simulink library "UXFD_Lib"  (R2016b)
settings: Solver=ode45  StartTime=0.0  StopTime=10.0  RelTol=1e-3  EnableMultiTasking=on
undefined symbols (not defined in the file): BreakpointData, BreakpointData1, BreakpointData2, BreakpointData_One_A, BreakpointData_Two_A, E2E_P01DataIDMode, E2E_P01ReceiverStatusType, EnumClass, iBit, initalValue, No_Runnable_Period, ObB_EidBsgStDerat_C, p_OVERRIDE_MASTER_SWITCH, SlDemoSign, SwitchOff_P, SwitchOn_P, Table, TableData_M, VCCTi33, VSysD_FidVehDerat1_C
libraries: simulink x28, CCMLib x11, UXFD_Lib x8, canmsglib x2, PTCC_Lib x1, hdlsllib x1
(part 2 of 7)

== system UXFD_Lib/Autosar/Dem_SetEventStatusDepPP ==
  VcEv : Inport
  EntryCond : EnablePort
  Dem_SetEventStatus : S-Function  FunctionName=Dem_SetEventStatusDep_flp  Parameters=dt  SFunctionDeploymentMode=off  EnableBusSupport=off  mask(TL_CustomCode){data={'#state',0,'#param',0,'#work',0,'#input',2,'codefile','Dem_SetEventStatusDep.c','prodcode',0,'logdata',{'plotchannels',[]},'output',{'name','$S_ok','varname','ok','type','Bool'},'input#1',{'name','$S_EventId','varname','EventId','type','UInt16'},'input#2',{'name','$S_EventStatus','varname','EventStatus','type','UInt8'},'date',735284.44087483792}, dt=-1}
      mask help:
      | TargetLink Custom Code block:
      | Allows to insert custom code into a TargetLink application.
      settings: AttributesFormatString=Dem_SetEventStatusDep  DeleteFcn=if exist('delete_tlblock','file')==2,delete_tlblock(gcbh);end  NameChangeFcn=if exist('rename_tlblock','file')==2,rename_tlblock(gcbh);end  OpenFcn=if exist('tl_open_blockdlg','file')==2,tl_open_blockdlg(gcbh);else,open_system(gcbh,'mask');end
      mask Help: eval(['tl_online_help(''Topic'',''',get_param(gcbh,'MaskType'),''')'])
      mask Display:
      | plot([-0.05, 1.05, NaN, -0.05, 1.05],[.01, .01, NaN, .99, .99])
      | ; disp('Dem_SetEventStatusDep.c');port_label('input',1,'EventId');port_label('input',2,'EventStatus');port_label('output',1,'ok');
  Pre-Passed : Constant  Value=2  mask(TL_Constant){data={'date',735284.44033693289}}
      settings: CopyFcn=if exist('tl_reset_reviewflag','file')==2,tl_reset_reviewflag(gcbh);end  DeleteFcn=if exist('delete_tlblock','file')==2,delete_tlblock(gcbh);end  NameChangeFcn=if exist('rename_tlblock','file')==2,rename_tlblock(gcbh);end  OpenFcn=if exist('tl_open_blockdlg','file')==2,tl_open_blockdlg(gcbh);else,open_system(gcbh,'parameter');end
      mask Help: eval(['if exist(''tl_online_help'',''file'') == 2, tl_online_help(''Topic'',''TL_Constant''),else, web([''jar:file:///'',matlabroot,''/help/toolbox/simulink/help.jar!/slref/' lower(get_param(gcbh,'Blocktype')) '.html''], ''-helpbrowser''),end'])
      mask Display: plot([-0.05, 1.05, NaN, -0.05, 1.05],[.01, .01, NaN, .99, .99])
  Terminator3 : Terminator
  wires:
  Dem_SetEventStatus/1 -> Terminator3/1
  VcEv/1 -> Dem_SetEventStatus/1
  Pre-Passed/1 -> Dem_SetEventStatus/2

== system UXFD_Lib/Autosar/Dem_SetEventStatusF ==
  VcEv : Inport
  EntryCond : EnablePort
  Dem_SetEventStatus : S-Function  FunctionName=Dem_SetEventStatus_flp  Parameters=dt  SFunctionDeploymentMode=off  EnableBusSupport=off  mask(TL_CustomCode){data={'#state',0,'#param',0,'#work',0,'#input',2,'codefile','Dem_SetEventStatus.c','prodcode',0,'logdata',{'plotchannels',[]},'output',{'name','$S_ok','varname','ok','type','Bool'},'input#1',{'name','$S_EventId','varname','EventId','type','UInt16'},'input#2',{'name','$S_EventStatus','varname','EventStatus','type','UInt8'},'date',735300.29239828698}, dt=-1}
      mask help:
      | TargetLink Custom Code block:
      | Allows to insert custom code into a TargetLink application.
      settings: AttributesFormatString=Dem_SetEventStatus  DeleteFcn=if exist('delete_tlblock','file')==2,delete_tlblock(gcbh);end  NameChangeFcn=if exist('rename_tlblock','file')==2,rename_tlblock(gcbh);end  OpenFcn=if exist('tl_open_blockdlg','file')==2,tl_open_blockdlg(gcbh);else,open_system(gcbh,'mask');end
      mask Help: eval(['tl_online_help(''Topic'',''',get_param(gcbh,'MaskType'),''')'])
      mask Display:
      | plot([-0.05, 1.05, NaN, -0.05, 1.05],[.01, .01, NaN, .99, .99])
      | ; disp('Dem_SetEventStatus.c');port_label('input',1,'EventId');port_label('input',2,'EventStatus');port_label('output',1,'ok');
  Failed : Constant  mask(TL_Constant){data={'date',735300.29239776626}}
      settings: CopyFcn=if exist('tl_reset_reviewflag','file')==2,tl_reset_reviewflag(gcbh);end  DeleteFcn=if exist('delete_tlblock','file')==2,delete_tlblock(gcbh);end  NameChangeFcn=if exist('rename_tlblock','file')==2,rename_tlblock(gcbh);end  OpenFcn=if exist('tl_open_blockdlg','file')==2,tl_open_blockdlg(gcbh);else,open_system(gcbh,'parameter');end
      mask Help: eval(['if exist(''tl_online_help'',''file'') == 2, tl_online_help(''Topic'',''TL_Constant''),else, web([''jar:file:///'',matlabroot,''/help/toolbox/simulink/help.jar!/slref/' lower(get_param(gcbh,'Blocktype')) '.html''], ''-helpbrowser''),end'])
      mask Display: plot([-0.05, 1.05, NaN, -0.05, 1.05],[.01, .01, NaN, .99, .99])
  Terminator3 : Terminator
  wires:
  Dem_SetEventStatus/1 -> Terminator3/1
  VcEv/1 -> Dem_SetEventStatus/1
  Failed/1 -> Dem_SetEventStatus/2

== system UXFD_Lib/Autosar/Dem_SetEventStatusP ==
  VcEv : Inport
  EntryCond : EnablePort
  Dem_SetEventStatus : S-Function  FunctionName=Dem_SetEventStatus_flp  Parameters=dt  SFunctionDeploymentMode=off  EnableBusSupport=off  mask(TL_CustomCode){data={'#state',0,'#param',0,'#work',0,'#input',2,'codefile','Dem_SetEventStatus.c','prodcode',0,'logdata',{'plotchannels',[]},'output',{'name','$S_ok','varname','ok','type','Bool'},'input#1',{'name','$S_EventId','varname','EventId','type','UInt16'},'input#2',{'name','$S_EventStatus','varname','EventStatus','type','UInt8'},'date',735300.29239747685}, dt=-1}
      mask help:
      | TargetLink Custom Code block:
      | Allows to insert custom code into a TargetLink application.
      settings: AttributesFormatString=Dem_SetEventStatus  DeleteFcn=if exist('delete_tlblock','file')==2,delete_tlblock(gcbh);end  NameChangeFcn=if exist('rename_tlblock','file')==2,rename_tlblock(gcbh);end  OpenFcn=if exist('tl_open_blockdlg','file')==2,tl_open_blockdlg(gcbh);else,open_system(gcbh,'mask');end
      mask Help: eval(['tl_online_help(''Topic'',''',get_param(gcbh,'MaskType'),''')'])
      mask Display:
      | plot([-0.05, 1.05, NaN, -0.05, 1.05],[.01, .01, NaN, .99, .99])
      | ; disp('Dem_SetEventStatus.c');port_label('input',1,'EventId');port_label('input',2,'EventStatus');port_label('output',1,'ok');
  Passed : Constant  Value=0  mask(TL_Constant){data={'date',735300.29239693284}}
      settings: CopyFcn=if exist('tl_reset_reviewflag','file')==2,tl_reset_reviewflag(gcbh);end  DeleteFcn=if exist('delete_tlblock','file')==2,delete_tlblock(gcbh);end  NameChangeFcn=if exist('rename_tlblock','file')==2,rename_tlblock(gcbh);end  OpenFcn=if exist('tl_open_blockdlg','file')==2,tl_open_blockdlg(gcbh);else,open_system(gcbh,'parameter');end
      mask Help: eval(['if exist(''tl_online_help'',''file'') == 2, tl_online_help(''Topic'',''TL_Constant''),else, web([''jar:file:///'',matlabroot,''/help/toolbox/simulink/help.jar!/slref/' lower(get_param(gcbh,'Blocktype')) '.html''], ''-helpbrowser''),end'])
      mask Display: plot([-0.05, 1.05, NaN, -0.05, 1.05],[.01, .01, NaN, .99, .99])
  Terminator3 : Terminator
  wires:
  Passed/1 -> Dem_SetEventStatus/2
  VcEv/1 -> Dem_SetEventStatus/1
  Dem_SetEventStatus/1 -> Terminator3/1

== system UXFD_Lib/Autosar/Dem_SetEventStatusPF ==
  VcEv : Inport
  EntryCond : EnablePort
  Dem_SetEventStatus : S-Function  FunctionName=Dem_SetEventStatus_flp  Parameters=dt  SFunctionDeploymentMode=off  EnableBusSupport=off  mask(TL_CustomCode){data={'#state',0,'#param',0,'#work',0,'#input',2,'codefile','Dem_SetEventStatus.c','prodcode',0,'logdata',{'plotchannels',[]},'output',{'name','$S_ok','varname','ok','type','Bool'},'input#1',{'name','$S_EventId','varname','EventId','type','UInt16'},'input#2',{'name','$S_EventStatus','varname','EventStatus','type','UInt8'},'date',735300.29239666671}, dt=-1}
      mask help:
      | TargetLink Custom Code block:
      | Allows to insert custom code into a TargetLink application.
      settings: AttributesFormatString=Dem_SetEventStatus  DeleteFcn=if exist('delete_tlblock','file')==2,delete_tlblock(gcbh);end  NameChangeFcn=if exist('rename_tlblock','file')==2,rename_tlblock(gcbh);end  OpenFcn=if exist('tl_open_blockdlg','file')==2,tl_open_blockdlg(gcbh);else,open_system(gcbh,'mask');end
      mask Help: eval(['tl_online_help(''Topic'',''',get_param(gcbh,'MaskType'),''')'])
      mask Display:
      | plot([-0.05, 1.05, NaN, -0.05, 1.05],[.01, .01, NaN, .99, .99])
      | ; disp('Dem_SetEventStatus.c');port_label('input',1,'EventId');port_label('input',2,'EventStatus');port_label('output',1,'ok');
  Pre-Failed : Constant  Value=3  mask(TL_Constant){data={'date',735300.2923961574}}
      settings: CopyFcn=if exist('tl_reset_reviewflag','file')==2,tl_reset_reviewflag(gcbh);end  DeleteFcn=if exist('delete_tlblock','file')==2,delete_tlblock(gcbh);end  NameChangeFcn=if exist('rename_tlblock','file')==2,rename_tlblock(gcbh);end  OpenFcn=if exist('tl_open_blockdlg','file')==2,tl_open_blockdlg(gcbh);else,open_system(gcbh,'parameter');end
      mask Help: eval(['if exist(''tl_online_help'',''file'') == 2, tl_online_help(''Topic'',''TL_Constant''),else, web([''jar:file:///'',matlabroot,''/help/toolbox/simulink/help.jar!/slref/' lower(get_param(gcbh,'Blocktype')) '.html''], ''-helpbrowser''),end'])
      mask Display: plot([-0.05, 1.05, NaN, -0.05, 1.05],[.01, .01, NaN, .99, .99])
  Terminator3 : Terminator
  wires:
  Pre-Failed/1 -> Dem_SetEventStatus/2
  VcEv/1 -> Dem_SetEventStatus/1
  Dem_SetEventStatus/1 -> Terminator3/1

== system UXFD_Lib/Autosar/Dem_SetEventStatusPP ==
  VcEv : Inport
  EntryCond : EnablePort
  Dem_SetEventStatus : S-Function  FunctionName=Dem_SetEventStatus_flp  Parameters=dt  SFunctionDeploymentMode=off  EnableBusSupport=off  mask(TL_CustomCode){data={'#state',0,'#param',0,'#work',0,'#input',2,'codefile','Dem_SetEventStatus.c','prodcode',0,'logdata',{'plotchannels',[]},'output',{'name','$S_ok','varname','ok','type','Bool'},'input#1',{'name','$S_EventId','varname','EventId','type','UInt16'},'input#2',{'name','$S_EventStatus','varname','EventStatus','type','UInt8'},'date',735300.29239586811}, dt=-1}
      mask help:
      | TargetLink Custom Code block:
      | Allows to insert custom code into a TargetLink application.
      settings: AttributesFormatString=Dem_SetEventStatus  DeleteFcn=if exist('delete_tlblock','file')==2,delete_tlblock(gcbh);end  NameChangeFcn=if exist('rename_tlblock','file')==2,rename_tlblock(gcbh);end  OpenFcn=if exist('tl_open_blockdlg','file')==2,tl_open_blockdlg(gcbh);else,open_system(gcbh,'mask');end
      mask Help: eval(['tl_online_help(''Topic'',''',get_param(gcbh,'MaskType'),''')'])
      mask Display:
      | plot([-0.05, 1.05, NaN, -0.05, 1.05],[.01, .01, NaN, .99, .99])
      | ; disp('Dem_SetEventStatus.c');port_label('input',1,'EventId');port_label('input',2,'EventStatus');port_label('output',1,'ok');
  Pre-Passed : Constant  Value=2  mask(TL_Constant){data={'date',735300.29237822921}}
      settings: CopyFcn=if exist('tl_reset_reviewflag','file')==2,tl_reset_reviewflag(gcbh);end  DeleteFcn=if exist('delete_tlblock','file')==2,delete_tlblock(gcbh);end  NameChangeFcn=if exist('rename_tlblock','file')==2,rename_tlblock(gcbh);end  OpenFcn=if exist('tl_open_blockdlg','file')==2,tl_open_blockdlg(gcbh);else,open_system(gcbh,'parameter');end
      mask Help: eval(['if exist(''tl_online_help'',''file'') == 2, tl_online_help(''Topic'',''TL_Constant''),else, web([''jar:file:///'',matlabroot,''/help/toolbox/simulink/help.jar!/slref/' lower(get_param(gcbh,'Blocktype')) '.html''], ''-helpbrowser''),end'])
      mask Display: plot([-0.05, 1.05, NaN, -0.05, 1.05],[.01, .01, NaN, .99, .99])
  Terminator3 : Terminator
  wires:
  Dem_SetEventStatus/1 -> Terminator3/1
  VcEv/1 -> Dem_SetEventStatus/1
  Pre-Passed/1 -> Dem_SetEventStatus/2

== system UXFD_Lib/Autosar/E2E_P01Protect ==
  DataLength : Inport
  DataID : Inport  Port=2
  Vmc_Out_BrkActrCtrlModForMinTqReq : Inport  Port=3
  Vmc_Out_BrkTqGrdtNegMinReq : Inport  Port=4
  Vmc_Out_BrkTqGrdtPosMinReq : Inport  Port=5
  Vmc_Out_BrkTqMinReq : Inport  Port=6
  E2E_P01Protect : Subsystem  TreatAsAtomicUnit=on
  Selector : Selector  InputPortWidth=9  IndexOptions=Index vector (dialog)  Indices=[1]  OutputSizes=1
  Selector1 : Selector  InputPortWidth=9  IndexOptions=Index vector (dialog)  Indices=[2]  OutputSizes=1
  Unit Delay1 : UnitDelay  SampleTime=-1
  Unit Delay2 : UnitDelay  SampleTime=-1
  E2E_P01Protect_ReturnType : Outport
  RollingCounter : Outport  Port=2
  CheckSum : Outport  Port=3
  wires:
  Selector/1 -> Unit Delay1/1, CheckSum/1
  Selector1/1 -> RollingCounter/1, Unit Delay2/1
  E2E_P01Protect/2(Data_pu8) -> Selector1/1, Selector/1
  DataLength/1 -> E2E_P01Protect/1(DataLength)
  DataID/1 -> E2E_P01Protect/2(DataID)
  E2E_P01Protect/1(E2E_P01Protect_ReturnType) -> E2E_P01Protect_ReturnType/1
  Unit Delay1/1 -> E2E_P01Protect/8(CheckSum_In)
  Unit Delay2/1 -> E2E_P01Protect/7(RollingCounter_In)
  Vmc_Out_BrkTqMinReq/1 -> E2E_P01Protect/6(Vmc_Out_BrkTqMinReq)
  Vmc_Out_BrkTqGrdtPosMinReq/1 -> E2E_P01Protect/5(Vmc_Out_BrkTqGrdtPosMinReq)
  Vmc_Out_BrkTqGrdtNegMinReq/1 -> E2E_P01Protect/4(Vmc_Out_BrkTqGrdtNegMinReq)
  Vmc_Out_BrkActrCtrlModForMinTqReq/1 -> E2E_P01Protect/3(Vmc_Out_BrkActrCtrlModForMinTqReq)

== system UXFD_Lib/Autosar/E2E_P01_Check ==
  AccrPedlNotCmpl_IsUpdated : Inport  OutDataTypeStr=boolean
  CheckSum : Inport  Port=2
  RollingCounter : Inport  Port=3
  AccrPedlNotCmpl_Psd : Inport  Port=4
  AccrPedlNotCmpl_PsdSts : Inport  Port=5
  DataID_ID : Constant  Value=205  OutDataTypeStr=uint16
  DataLength : Constant  Value=32  OutDataTypeStr=uint16
  E2E_Check : Subsystem
  E2E_check_OK : Outport
  wires:
  DataLength/1 -> E2E_Check/1(DataLength)
  DataID_ID/1 -> E2E_Check/2(DataID)
  AccrPedlNotCmpl_IsUpdated/1 -> E2E_Check/3(AccrPedlNotCmpl_IsUpdated)
  CheckSum/1 -> E2E_Check/4(CheckSum)
  RollingCounter/1 -> E2E_Check/5(RollingCounter)
  E2E_Check/1(CRC_Valid) -> E2E_check_OK/1
  AccrPedlNotCmpl_Psd/1 -> E2E_Check/6(AccrPedlNotCmpl_Psd)
  AccrPedlNotCmpl_PsdSts/1 -> E2E_Check/7(AccrPedlNotCmpl_PsdSts)

== system UXFD_Lib/Autosar/FiM_GetFunctionPermission ==
  note: A fix for setting the correct data type in simulink.
      | The data type set in TL does not seem to propagete to
      | the simulink block.
  VcFi : Inport
  EntryCond : EnablePort
  Data Type Conversion : DataTypeConversion  OutDataTypeStr=boolean
  FiM_GetFunctionPermission : S-Function  Description=I: FID, O1 = ok, O2 = Permission  FunctionName=FiM_GetFunctionPermission_flp  Parameters=dt  SFunctionDeploymentMode=off  EnableBusSupport=off  mask(TL_CustomCode){data={'#state',0,'#param',0,'#work',0,'#output',2,'#logdata',2,'codefile','FiM_GetFunctionPermission.c','prodcode',0,'logdata#1',{'plotchannels',[]},'logdata#2',{'plotchannels',[]},'output#1',{'name','$S_ok','varname','ok','type','Bool'},'output#2',{'name','$S_perm','varname','permission','type','Bool'},'input',{'name','$S_FID','varname','FID','type','UInt16'},'date',736012.81500542827}, dt=-1}
      mask help:
      | TargetLink Custom Code block:
      | Allows to insert custom code into a TargetLink application.
      settings: AttributesFormatString=FiM_GetFunctionPermission  DeleteFcn=if exist('delete_tlblock','file')==2,delete_tlblock(gcbh);end  NameChangeFcn=if exist('rename_tlblock','file')==2,rename_tlblock(gcbh);end  OpenFcn=if exist('tl_open_blockdlg','file')==2,tl_open_blockdlg(gcbh);else,open_system(gcbh,'mask');end
      mask Help: eval(['tl_online_help(''Topic'',''',get_param(gcbh,'MaskType'),''')'])
      mask Display:
      | plot([-0.05, 1.05, NaN, -0.05, 1.05],[.01, .01, NaN, .99, .99])
      | ; disp('FiM_GetFunctionPermission.c');port_label('input',1,'FID');port_label('output',1,'ok');port_label('output',2,'permission');
  Terminator4 : Terminator
  Perm : Outport
  wires:
  FiM_GetFunctionPermission/2 -> Data Type Conversion/1
  FiM_GetFunctionPermission/1 -> Terminator4/1
  VcFi/1 -> FiM_GetFunctionPermission/1
  Data Type Conversion/1 -> Perm/1

== system UXFD_Lib/Autosar/NamedConstant ==
  Constant : Constant  Value=0  mask(TL_Constant){data={'output',{'name','$E(const_name)','class','EXTERN_GLOBAL_ALIAS','type','UInt16'},'date',735602.50771956018}}
      settings: AttributesFormatString=%<const_name>  CopyFcn=if exist('tl_reset_reviewflag') == 2, tl_reset_reviewflag(gcbh); end  DeleteFcn=if exist('delete_tlblock','file')==2,delete_tlblock(gcbh);end  NameChangeFcn=if exist('rename_tlblock','file')==2,rename_tlblock(gcbh);end  OpenFcn=if exist('tl_open_blockdlg','file')==2,tl_open_blockdlg(gcbh);else,open_system(gcbh,'parameter');end
      mask Help: eval(['if exist(''tl_online_help'',''file'') == 2, tl_online_help(''Topic'',''TL_Constant''),else, web([''jar:file:///'',matlabroot,''/help/toolbox/simulink/help.jar!/slref/' lower(get_param(gcbh,'Blocktype')) '.html''], ''-helpbrowser''),end'])
      mask Display: plot([-0.05, 1.05, NaN, -0.05, 1.05],[.01, .01, NaN, .99, .99])
  Perm : Outport
  wires:
  Constant/1 -> Perm/1

== system UXFD_Lib/Autosar/xbackground4 ==

== system UXFD_Lib/Autosar/xbackground5 ==

== system UXFD_Lib/CCM/1-D LookupTable ==
  XAxis : Inport
  1-D Lookup Table : Lookup_n-D  NumberOfTableDimensions=1  BreakpointsForDimension1=BreakpointsXAxis  BreakpointsForDimension1DataTypeStr=BreakpointsXAxisDataType  Table=TableData  TableDataTypeStr=TableDataDataType  ExtrapMethod=Clip  UseLastTableValue=on  OutDataTypeStr=TableDataDataType  SaturateOnIntegerOverflow=on
  Out : Outport
  wires:
  1-D Lookup Table/1 -> Out/1
  XAxis/1 -> 1-D Lookup Table/1

== system UXFD_Lib/CCM/2-D LookupTable ==
  XAxis : Inport
  YAxis : Inport  Port=2
  2-D Lookup Table : Lookup_n-D  BreakpointsForDimension1=BreakpointsYAxis  BreakpointsForDimension2=BreakpointsXAxis  BreakpointsForDimension1DataTypeStr=BreakpointsYAxisDataType  BreakpointsForDimension2DataTypeStr=BreakpointsXAxisDataType  Table=TableData  TableDataTypeStr=TableDataDataType  ExtrapMethod=Clip  UseLastTableValue=on  OutDataTypeStr=TableDataDataType  SaturateOnIntegerOverflow=on
  Out : Outport
  wires:
  XAxis/1 -> 2-D Lookup Table/2
  YAxis/1 -> 2-D Lookup Table/1
  2-D Lookup Table/1 -> Out/1

== system UXFD_Lib/CCM/CompareToEnum ==
  u : Inport
  Compare : RelationalOperator  Operator===  OutDataTypeStr=boolean  RndMeth=Nearest  InputSameDT=on
  Constant : Constant  DisableCoverage=on  Value=const  OutDataTypeStr=Inherit: Inherit via back propagation
  y : Outport
  wires:
  u/1 -> Compare/1
  Constant/1 -> Compare/2
  Compare/1 -> y/1

== system UXFD_Lib/CCM/Conversion ==
  In : Inport
  Data Type Conversion : DataTypeConversion  OutDataTypeStr=outputDataType  SaturateOnIntegerOverflow=on
  Out : Outport
  wires:
  In/1 -> Data Type Conversion/1
  Data Type Conversion/1 -> Out/1

== system UXFD_Lib/CCM/Counter ==
  note: CounterRunning
  Start : Inport  OutDataTypeStr=boolean
  Reset : Inport  Port=2  OutDataTypeStr=boolean
  IC : Constant  Value=0  OutDataTypeStr=VCCUInt32  SampleTime=-1
  Increment : Constant  OutDataTypeStr=VCCUInt32  SampleTime=-1
  Logical Operator : Logic  AllPortsSameDT=off  OutDataTypeStr=boolean
  Logical Operator1 : Logic  Operator=NOT  AllPortsSameDT=off  OutDataTypeStr=boolean
  Logical Operator2 : Logic  Operator=OR  AllPortsSameDT=off  OutDataTypeStr=boolean
  StopCounter : Constant  Value=0  OutDataTypeStr=VCCUInt32  SampleTime=-1
  Sum : Sum  OutDataTypeStr=VCCUInt32  SaturateOnIntegerOverflow=on
  Switch : Switch  Criteria=u2 ~= 0  SaturateOnIntegerOverflow=on
  Unit Delay External IC : simulink/Additional Math & Discrete/Additional Discrete/Unit Delay External IC  tsamp=-1
  Unit Delay Resettable External IC : CCMLib/Unit Delay Resettable External IC  dataType=VCCUInt32
  false : Constant  Value=false  OutDataTypeStr=boolean  SampleTime=-1
  Value : Outport  OutDataTypeStr=VCCUInt32
  wires:
  StopCounter/1 -> Switch/3
  Increment/1 -> Switch/1
  Switch/1 -> Sum/2
  Reset/1 -> Unit Delay Resettable External IC/3, Logical Operator1/1
  Sum/1 -> Unit Delay Resettable External IC/1
  Unit Delay Resettable External IC/1 -> Value/1, Sum/1
  IC/1 -> Unit Delay Resettable External IC/2
  Unit Delay External IC/1 -> Logical Operator2/1
  Start/1 -> Logical Operator2/2
  Logical Operator/1 -> Unit Delay External IC/1, Switch/2
  false/1 -> Unit Delay External IC/2
  Logical Operator2/1 -> Logical Operator/1
  Logical Operator1/1 -> Logical Operator/2

== system UXFD_Lib/CCM/Counter Holdable ==
  note: CounterRunning
  Start : Inport  OutDataTypeStr=boolean
  Hold : Inport  Port=2  OutDataTypeStr=boolean
  Reset : Inport  Port=3  OutDataTypeStr=boolean
  IC : Constant  Value=0  OutDataTypeStr=VCCUInt32  SampleTime=-1
  Increment : Constant  OutDataTypeStr=VCCUInt32  SampleTime=-1
  Logical Operator : Logic  AllPortsSameDT=off  OutDataTypeStr=boolean
  Logical Operator1 : Logic  Operator=NOT  AllPortsSameDT=off  OutDataTypeStr=boolean
  Logical Operator2 : Logic  Operator=OR  AllPortsSameDT=off  OutDataTypeStr=boolean
  StopCounter : Constant  Value=0  OutDataTypeStr=VCCUInt32  SampleTime=-1
  Sum : Sum  OutDataTypeStr=VCCUInt32  SaturateOnIntegerOverflow=on
  Switch : Switch  Criteria=u2 ~= 0  SaturateOnIntegerOverflow=on
  Unit Delay External IC : simulink/Additional Math & Discrete/Additional Discrete/Unit Delay External IC  tsamp=-1
  Unit Delay Resettable External IC1 : CCMLib/Unit Delay Resettable External IC  dataType=VCCUInt32
  false : Constant  Value=false  OutDataTypeStr=boolean  SampleTime=-1
  Value : Outport  OutDataTypeStr=VCCUInt32
  wires:
  IC/1 -> Unit Delay Resettable External IC1/2
  Unit Delay Resettable External IC1/1 -> Sum/1, Value/1
  Sum/1 -> Unit Delay Resettable External IC1/1
  Logical Operator1/1 -> Logical Operator/2
  Hold/1 -> Logical Operator1/1
  Logical Operator2/1 -> Logical Operator/1
  false/1 -> Unit Delay External IC/2
  Logical Operator/1 -> Switch/2, Unit Delay External IC/1
  Start/1 -> Logical Operator2/2
  Unit Delay External IC/1 -> Logical Operator2/1
  Reset/1 -> Unit Delay Resettable External IC1/3
  Switch/1 -> Sum/2
  Increment/1 -> Switch/1
  StopCounter/1 -> Switch/3

== system UXFD_Lib/CCM/LowPass filter ==
  note: filtered signal
  note: NOTE!
      | LPF_Time_Constant must be greater
      | or equal to the Sample_Time
  U : Inport  OutDataTypeStr=InputOutputDataType
  FilCon : Inport  Port=2  OutDataTypeStr=FilterConstantDataType
  Constant : Constant  OutDataTypeStr=single  SampleTime=-1
  Data Type Conversion1 : DataTypeConversion  OutDataTypeStr=single  RndMeth=Round  SaturateOnIntegerOverflow=on
  MinMax : MinMax  Function=max  Inputs=2  OutDataTypeStr=single  SaturateOnIntegerOverflow=on
  OutputDataType : DataTypeConversion  OutDataTypeStr=InputOutputDataType  RndMeth=Round  SaturateOnIntegerOverflow=on
  Product1 : Product  Inputs=*/  OutDataTypeStr=single  SaturateOnIntegerOverflow=on
  Product2 : Product  OutDataTypeStr=single  SaturateOnIntegerOverflow=on
  Product3 : Product  OutDataTypeStr=single  SaturateOnIntegerOverflow=on
  RunnablePeriod : Constant  Value=RunnablePeriod  OutDataTypeStr=single  SampleTime=-1
  Sum : Sum  Inputs=+-  OutDataTypeStr=single  SaturateOnIntegerOverflow=on
  Sum1 : Sum  OutDataTypeStr=single  SaturateOnIntegerOverflow=on
  Unit Delay External IC : CCMLib/Unit Delay External IC  dataType=single
  Y : Outport  OutDataTypeStr=InputOutputDataType
  wires:
  FilCon/1 -> MinMax/2
  MinMax/1 -> Product1/2
  OutputDataType/1 -> Y/1
  U/1 -> Data Type Conversion1/1
  RunnablePeriod/1 -> MinMax/1, Product1/1
  Product2/1 -> Sum1/2
  Sum1/1 -> Unit Delay External IC/1, OutputDataType/1
  Unit Delay External IC/1 -> Product2/2
  Product3/1 -> Sum1/1
  Sum/1 -> Product2/1
  Product1/1 -> Product3/2, Sum/2
  Data Type Conversion1/1 -> Unit Delay External IC/2, Product3/1
  Constant/1 -> Sum/1

== system UXFD_Lib/CCM/LowPass filter Resettable ==
  note: NOTE!
      | LPF_Time_Constant must be greater
      | or equal to the Sample_Time
  note: filtered signal
  U : Inport  OutDataTypeStr=InputOutputDataType
  FilCon : Inport  Port=2  OutDataTypeStr=FilterConstantDataType
  Rst : Inport  Port=3  OutDataTypeStr=boolean
  Constant : Constant  OutDataTypeStr=single  SampleTime=-1
  Data Type Conversion1 : DataTypeConversion  OutDataTypeStr=single  SaturateOnIntegerOverflow=on
  MinMax : MinMax  Function=max  Inputs=2  OutDataTypeStr=single  SaturateOnIntegerOverflow=on
  OutputDataType : DataTypeConversion  OutDataTypeStr=InputOutputDataType  RndMeth=Round  SaturateOnIntegerOverflow=on
  Product1 : Product  Inputs=*/  OutDataTypeStr=single  SaturateOnIntegerOverflow=on  RndMeth=Zero
  Product2 : Product  OutDataTypeStr=single  SaturateOnIntegerOverflow=on
  Product3 : Product  OutDataTypeStr=single  SaturateOnIntegerOverflow=on
  RunnablePeriod : Constant  Value=RunnablePeriod  OutDataTypeStr=single  SampleTime=-1
  Sum : Sum  Inputs=+-  OutDataTypeStr=single  SaturateOnIntegerOverflow=on
  Sum1 : Sum  OutDataTypeStr=single  SaturateOnIntegerOverflow=on
  Unit Delay Resettable External IC boolean controlled : Subsystem  mask(Unit Delay Resettable External Initial Condition (boolean)){dt=single, UnitDelayInitCondition=0}
      mask prompts: dt "Data type in/out"; UnitDelayInitCondition "Internal unit delay block initial condition:"
      mask help:
      | This is the same block as the Simulink standard, except all fix point
      | data-types have been changed to booleans.
      | The internal unit delay block can often be kept as 0, unless the input/output signal is of ENUM type.
      | Made by Niklas Magnusson (nmagnus3).
      | NGCC
      mask Display: dpoly(1,[1 0],'z')
  Y : Outport  OutDataTypeStr=InputOutputDataType
  wires:
  Constant/1 -> Sum/1
  Data Type Conversion1/1 -> Product3/1, Unit Delay Resettable External IC boolean controlled/3(IC)
  Product1/1 -> Sum/2, Product3/2
  Sum/1 -> Product2/1
  Product3/1 -> Sum1/1
  Unit Delay Resettable External IC boolean controlled/1(y) -> Product2/2
  Sum1/1 -> OutputDataType/1, Unit Delay Resettable External IC boolean controlled/1(u)
  Product2/1 -> Sum1/2
  RunnablePeriod/1 -> Product1/1, MinMax/1
  U/1 -> Data Type Conversion1/1
  OutputDataType/1 -> Y/1
  Rst/1 -> Unit Delay Resettable External IC boolean controlled/2(R)
  MinMax/1 -> Product1/2
  FilCon/1 -> MinMax/2

== system UXFD_Lib/CCM/LowPass filter IC ==
  note: filtered signal
  note: NOTE!
      | LPF_Time_Constant must be greater
      | or equal to the Sample_Time
  U : Inport  OutDataTypeStr=InputOutputDataType
  IC : Inport  Port=2  OutDataTypeStr=InputOutputDataType
  FilCon : Inport  Port=3  OutDataTypeStr=FilterConstantDataType
  Constant : Constant  OutDataTypeStr=single  SampleTime=-1
  Data Type Conversion1 : DataTypeConversion  OutDataTypeStr=single  RndMeth=Round  SaturateOnIntegerOverflow=on
  Data Type Conversion2 : DataTypeConversion  OutDataTypeStr=single  RndMeth=Round  SaturateOnIntegerOverflow=on
  EnableIC : Constant  Value=true  OutDataTypeStr=boolean  SampleTime=-1
  MinMax : MinMax  Function=max  Inputs=2  OutDataTypeStr=single  SaturateOnIntegerOverflow=on
  OutputDataType : DataTypeConversion  OutDataTypeStr=InputOutputDataType  RndMeth=Round  SaturateOnIntegerOverflow=on
  Product1 : Product  Inputs=*/  OutDataTypeStr=single  SaturateOnIntegerOverflow=on
  Product2 : Product  OutDataTypeStr=single  SaturateOnIntegerOverflow=on
  Product3 : Product  OutDataTypeStr=single  SaturateOnIntegerOverflow=on
  RunnablePeriod : Constant  Value=RunnablePeriod  OutDataTypeStr=single  SampleTime=-1
  Sum : Sum  Inputs=+-  OutDataTypeStr=single  SaturateOnIntegerOverflow=on
  Sum1 : Sum  OutDataTypeStr=single  SaturateOnIntegerOverflow=on
  Switch : Switch  Criteria=u2 ~= 0  SaturateOnIntegerOverflow=on
  Unit Delay : UnitDelay  InitialCondition=false  SampleTime=-1
      settings: AttributesFormatString=X0=%<X0>
  Unit Delay External IC : CCMLib/Unit Delay External IC  dataType=single
  Y : Outport  OutDataTypeStr=InputOutputDataType
  wires:
  EnableIC/1 -> Unit Delay/1
  Unit Delay/1 -> Switch/2
  Switch/1 -> OutputDataType/1
  FilCon/1 -> MinMax/2
  MinMax/1 -> Product1/2
  OutputDataType/1 -> Y/1
  U/1 -> Data Type Conversion1/1
  RunnablePeriod/1 -> MinMax/1, Product1/1
  Product2/1 -> Sum1/2
  Sum1/1 -> Switch/1, Unit Delay External IC/1
  Unit Delay External IC/1 -> Product2/2
  Product3/1 -> Sum1/1
  Sum/1 -> Product2/1
  Product1/1 -> Product3/2, Sum/2
  Data Type Conversion1/1 -> Product3/1
  Constant/1 -> Sum/1
  IC/1 -> Data Type Conversion2/1
  Data Type Conversion2/1 -> Switch/3, Unit Delay External IC/2

== system UXFD_Lib/CCM/LowPass filter IC Resettable ==
  note: filtered signal
  note: NOTE!
      | LPF_Time_Constant must be greater
      | or equal to the Sample_Time
  U : Inport  OutDataTypeStr=InputOutputDataType
  IC : Inport  Port=2  OutDataTypeStr=InputOutputDataType
  FilCon : Inport  Port=3  OutDataTypeStr=FilterConstantDataType
  Rst : Inport  Port=4  OutDataTypeStr=boolean
  Constant : Constant  OutDataTypeStr=single  SampleTime=-1
  Data Type Conversion1 : DataTypeConversion  OutDataTypeStr=single  SaturateOnIntegerOverflow=on
  Data Type Conversion2 : DataTypeConversion  OutDataTypeStr=single  SaturateOnIntegerOverflow=on
  DisableIC : Constant  Value=false  OutDataTypeStr=boolean  SampleTime=-1
  Logical Operator : Logic  Operator=OR  AllPortsSameDT=off  OutDataTypeStr=boolean
  MinMax : MinMax  Function=max  Inputs=2  OutDataTypeStr=single  SaturateOnIntegerOverflow=on
  OutputDataType : DataTypeConversion  OutDataTypeStr=InputOutputDataType  RndMeth=Round  SaturateOnIntegerOverflow=on
  Product1 : Product  Inputs=*/  OutDataTypeStr=single  SaturateOnIntegerOverflow=on  RndMeth=Zero
  Product2 : Product  OutDataTypeStr=single  SaturateOnIntegerOverflow=on
  Product3 : Product  OutDataTypeStr=single  SaturateOnIntegerOverflow=on
  RunnablePeriod : Constant  Value=RunnablePeriod  OutDataTypeStr=single  SampleTime=-1
  Sum : Sum  Inputs=+-  OutDataTypeStr=single  SaturateOnIntegerOverflow=on
  Sum1 : Sum  OutDataTypeStr=single  SaturateOnIntegerOverflow=on
  Switch : Switch  Criteria=u2 ~= 0  SaturateOnIntegerOverflow=on
  Unit Delay : UnitDelay  InitialCondition=true  SampleTime=-1
      settings: AttributesFormatString=X0=%<X0>
  Unit Delay Resettable External IC boolean controlled : Subsystem  mask(Unit Delay Resettable External Initial Condition (boolean)){dt=single, UnitDelayInitCondition=0}
      mask prompts: dt "Data type in/out"; UnitDelayInitCondition "Internal unit delay block initial condition:"
      mask help:
      | This is the same block as the Simulink standard, except all fix point
      | data-types have been changed to booleans.
      | The internal unit delay block can often be kept as 0, unless the input/output signal is of ENUM type.
      | Made by Niklas Magnusson (nmagnus3).
      | NGCC
      mask Display: dpoly(1,[1 0],'z')
  Y : Outport  OutDataTypeStr=InputOutputDataType
  wires:
  Logical Operator/1 -> Switch/2
  Unit Delay/1 -> Logical Operator/1
  DisableIC/1 -> Unit Delay/1
  Switch/1 -> OutputDataType/1
  Data Type Conversion2/1 -> Switch/1, Unit Delay Resettable External IC boolean controlled/3(IC)
  IC/1 -> Data Type Conversion2/1
  FilCon/1 -> MinMax/2
  MinMax/1 -> Product1/2
  Rst/1 -> Logical Operator/2, Unit Delay Resettable External IC boolean controlled/2(R)
  OutputDataType/1 -> Y/1
  U/1 -> Data Type Conversion1/1
  RunnablePeriod/1 -> MinMax/1, Product1/1
  Product2/1 -> Sum1/2
  Sum1/1 -> Switch/3, Unit Delay Resettable External IC boolean controlled/1(u)
  Unit Delay Resettable External IC boolean controlled/1(y) -> Product2/2
  Product3/1 -> Sum1/1
  Sum/1 -> Product2/1
  Product1/1 -> Product3/2, Sum/2
  Data Type Conversion1/1 -> Product3/1
  Constant/1 -> Sum/1

== system UXFD_Lib/CCM/NonZero Division ==
  note: Data type conversion blocks are used to avoid error
      | when using unary minus on an unsigned data type.
  num : Inport  OutDataTypeStr=dataTypeNum
  denom : Inport  Port=2  OutDataTypeStr=dataTypeDen
  Constant1 : Constant  Value=0  OutDataTypeStr=dataTypeDen  SampleTime=-1
  Constant2 : Constant  Value=dataTypeSlope  OutDataTypeStr=dataTypeDen  SampleTime=-1
  Conversion2 : CCMLib/Conversion  outputDataType=single
  Conversion3 : CCMLib/Conversion  outputDataType=dataTypeDen
  Divide : Product  Inputs=*/  OutDataTypeStr=dataTypeOut  SaturateOnIntegerOverflow=on  RndMeth=Zero
  MinMax : MinMax  Inputs=2  OutDataTypeStr=dataTypeDen  RndMeth=Zero  SaturateOnIntegerOverflow=on
  MinMax1 : MinMax  Function=max  Inputs=2  OutDataTypeStr=dataTypeDen  RndMeth=Zero  SaturateOnIntegerOverflow=on
  Relational Operator1 : RelationalOperator  OutDataTypeStr=boolean  RndMeth=Nearest
  Switch2 : Switch  Criteria=u2 ~= 0  RndMeth=Zero  SaturateOnIntegerOverflow=on
  Unary Minus1 : UnaryMinus  SaturateOnIntegerOverflow=on
  y : Outport  OutDataTypeStr=dataTypeOut
  wires:
  Conversion3/1 -> MinMax/2
  Switch2/1 -> Divide/2
  Conversion2/1 -> Unary Minus1/1
  Constant2/1 -> MinMax1/2, Conversion2/1
  Unary Minus1/1 -> Conversion3/1
  MinMax/1 -> Switch2/3
  MinMax1/1 -> Switch2/1
  Relational Operator1/1 -> Switch2/2
  Constant1/1 -> Relational Operator1/2
  Divide/1 -> y/1
  denom/1 -> MinMax/1, MinMax1/1, Relational Operator1/1
  num/1 -> Divide/1

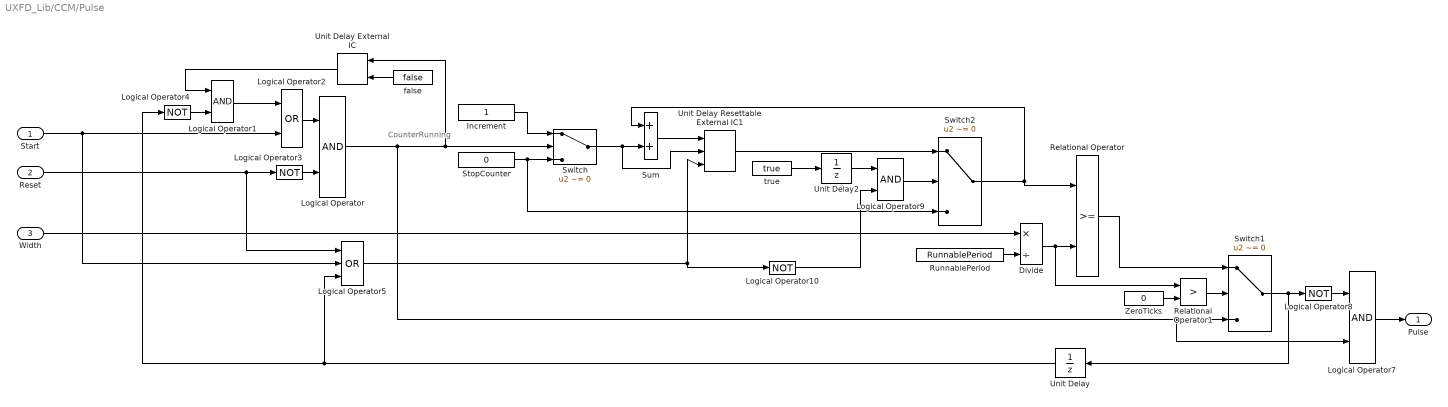
== system UXFD_Lib/CCM/Pulse ==
  note: CounterRunning
  Start : Inport  OutDataTypeStr=boolean
  Reset : Inport  Port=2  OutDataTypeStr=boolean
  Width : Inport  Port=3  OutDataTypeStr=timeDataType
  Divide : Product  Inputs=*/  OutDataTypeStr=VCCUInt32  RndMeth=Round  SaturateOnIntegerOverflow=on
  Increment : Constant  OutDataTypeStr=VCCUInt32  SampleTime=-1
  Logical Operator{,1,7,9} (4 alike) : Logic  AllPortsSameDT=off  OutDataTypeStr=boolean
  Logical Operator{3..4,8,10} (4 alike) : Logic  Operator=NOT  AllPortsSameDT=off  OutDataTypeStr=boolean
  Logical Operator2 : Logic  Operator=OR  AllPortsSameDT=off  OutDataTypeStr=boolean
  Logical Operator5 : Logic  Operator=OR  Inputs=3  AllPortsSameDT=off  OutDataTypeStr=boolean
  Relational Operator : RelationalOperator  OutDataTypeStr=boolean  RndMeth=Nearest
  Relational Operator1 : RelationalOperator  Operator=>  OutDataTypeStr=boolean  RndMeth=Nearest
  RunnablePeriod : Constant  Value=RunnablePeriod  OutDataTypeStr=VCCTiSamplePerd  SampleTime=-1
  StopCounter : Constant  Value=0  OutDataTypeStr=VCCUInt32  SampleTime=-1
  Sum : Sum  OutDataTypeStr=VCCUInt32  SaturateOnIntegerOverflow=on
  Switch : Switch  Criteria=u2 ~= 0  SaturateOnIntegerOverflow=on
  Switch1 : Switch  Criteria=u2 ~= 0  SaturateOnIntegerOverflow=on
  Switch2 : Switch  Criteria=u2 ~= 0  SaturateOnIntegerOverflow=on
  Unit Delay : UnitDelay  InitialCondition=false  SampleTime=-1
      settings: AttributesFormatString=X0=%<X0>
  Unit Delay External IC : simulink/Additional Math & Discrete/Additional Discrete/Unit Delay External IC  tsamp=-1
  Unit Delay Resettable External IC1 : CCMLib/Unit Delay Resettable External IC  dataType=VCCUInt32
  Unit Delay2 : UnitDelay  InitialCondition=false  SampleTime=-1
      settings: AttributesFormatString=X0=%<X0>
  ZeroTicks : Constant  Value=0  OutDataTypeStr=VCCUInt32  SampleTime=-1
  false : Constant  Value=false  OutDataTypeStr=boolean  SampleTime=-1
  true : Constant  Value=true  OutDataTypeStr=boolean  SampleTime=-1
  Pulse : Outport  OutDataTypeStr=boolean
  wires:
  Logical Operator4/1 -> Logical Operator1/2
  Logical Operator1/1 -> Logical Operator2/1
  Logical Operator7/1 -> Pulse/1
  Logical Operator8/1 -> Logical Operator7/1
  Start/1 -> Logical Operator5/2, Logical Operator2/2
  Unit Delay/1 -> Logical Operator4/1, Logical Operator5/3
  Reset/1 -> Logical Operator5/1, Logical Operator3/1
  Switch1/1 -> Logical Operator8/1, Unit Delay/1
  Logical Operator2/1 -> Logical Operator/1
  false/1 -> Unit Delay External IC/2
  Logical Operator/1 -> Switch/2, Unit Delay External IC/1, Logical Operator7/2, Switch1/3
  Unit Delay External IC/1 -> Logical Operator1/1
  Switch/1 -> Sum/2, Unit Delay Resettable External IC1/2
  Increment/1 -> Switch/1
  StopCounter/1 -> Switch/3, Switch2/3
  RunnablePeriod/1 -> Divide/2
  ZeroTicks/1 -> Relational Operator1/2
  Relational Operator1/1 -> Switch1/2
  Relational Operator/1 -> Switch1/1
  Divide/1 -> Relational Operator/2, Relational Operator1/1
  Logical Operator3/1 -> Logical Operator/2
  Width/1 -> Divide/1
  Sum/1 -> Unit Delay Resettable External IC1/1
  Logical Operator5/1 -> Unit Delay Resettable External IC1/3, Logical Operator10/1
  Unit Delay Resettable External IC1/1 -> Switch2/1
  true/1 -> Unit Delay2/1
  Logical Operator9/1 -> Switch2/2
  Unit Delay2/1 -> Logical Operator9/1
  Logical Operator10/1 -> Logical Operator9/2
  Switch2/1 -> Relational Operator/1, Sum/1

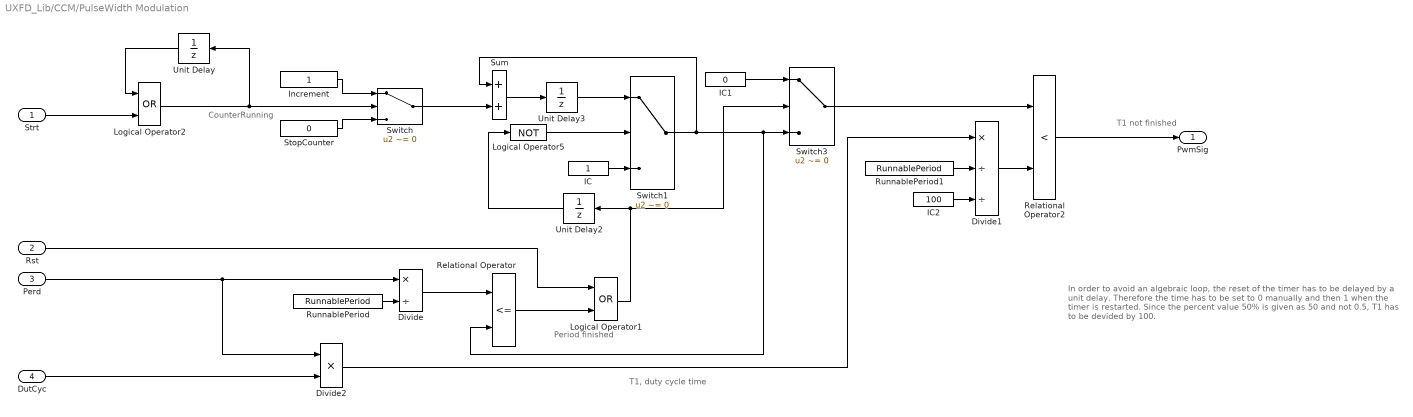
== system UXFD_Lib/CCM/PulseWidth Modulation ==
  note: T1, duty cycle time
  note: In order to avoid an algebraic loop, the reset of the timer has to be
      | delayed by a unit delay. Therefore the time has to be set to 0 manually
      | and then 1 when the timer is restarted.
      | Since the percent value 50% is given as 50 and not 0.5, T1 has to be
      | devided by 100.
  note: CounterRunning
  note: Period finished
  note: T1 not finished
  Strt : Inport  OutDataTypeStr=boolean
  Rst : Inport  Port=2  OutDataTypeStr=boolean
  Perd : Inport  Port=3  OutDataTypeStr=timeDataType
  DutCyc : Inport  Port=4  OutDataTypeStr=VCCPerc30
  Divide : Product  Inputs=*/  OutDataTypeStr=VCCUInt32  RndMeth=Round  SaturateOnIntegerOverflow=on
  Divide1 : Product  Inputs=*//  OutDataTypeStr=VCCUInt32  RndMeth=Round  SaturateOnIntegerOverflow=on
  Divide2 : Product  Inputs=**  OutDataTypeStr=VCCTi33  RndMeth=Round  SaturateOnIntegerOverflow=on
  IC : Constant  OutDataTypeStr=VCCUInt32  SampleTime=-1
  IC1 : Constant  Value=0  OutDataTypeStr=VCCUInt32  SampleTime=-1
  IC2 : Constant  Value=100  OutDataTypeStr=VCCUInt32  SampleTime=-1
  Increment : Constant  OutDataTypeStr=VCCUInt32  SampleTime=-1
  Logical Operator1 : Logic  Operator=OR  AllPortsSameDT=off  OutDataTypeStr=boolean
  Logical Operator2 : Logic  Operator=OR  AllPortsSameDT=off  OutDataTypeStr=boolean
  Logical Operator5 : Logic  Operator=NOT  Inputs=1  AllPortsSameDT=off  OutDataTypeStr=boolean
  Relational Operator : RelationalOperator  Operator=<=  OutDataTypeStr=boolean  RndMeth=Nearest
  Relational Operator2 : RelationalOperator  Operator=<  OutDataTypeStr=boolean  RndMeth=Nearest
  RunnablePeriod : Constant  Value=RunnablePeriod  OutDataTypeStr=VCCTiSamplePerd  SampleTime=-1
  RunnablePeriod1 : Constant  Value=RunnablePeriod  OutDataTypeStr=VCCTiSamplePerd  SampleTime=-1
  StopCounter : Constant  Value=0  OutDataTypeStr=VCCUInt32  SampleTime=-1
  Sum : Sum  OutDataTypeStr=VCCUInt32  SaturateOnIntegerOverflow=on
  Switch : Switch  Criteria=u2 ~= 0  SaturateOnIntegerOverflow=on
  Switch1 : Switch  Criteria=u2 ~= 0  SaturateOnIntegerOverflow=on
  Switch3 : Switch  Criteria=u2 ~= 0  SaturateOnIntegerOverflow=on
  Unit Delay : UnitDelay  InitialCondition=false  SampleTime=-1
      settings: AttributesFormatString=X0=%<X0>
  Unit Delay2 : UnitDelay  InitialCondition=false  SampleTime=-1
      settings: AttributesFormatString=X0=%<X0>
  Unit Delay3 : UnitDelay  SampleTime=-1
      settings: AttributesFormatString=X0=%<X0>
  PwmSig : Outport  OutDataTypeStr=boolean
  wires:
  Relational Operator2/1 -> PwmSig/1
  Unit Delay2/1 -> Logical Operator5/1
  Logical Operator1/1 -> Switch3/2, Unit Delay2/1
  Rst/1 -> Logical Operator1/1
  Relational Operator/1 -> Logical Operator1/2
  IC2/1 -> Divide1/3
  IC/1 -> Switch1/3
  Logical Operator5/1 -> Switch1/2
  Switch1/1 -> Relational Operator/2, Switch3/3, Sum/1
  Unit Delay3/1 -> Switch1/1
  Sum/1 -> Unit Delay3/1
  Divide2/1 -> Divide1/1
  RunnablePeriod1/1 -> Divide1/2
  DutCyc/1 -> Divide2/2
  Divide/1 -> Relational Operator/1
  Switch3/1 -> Relational Operator2/1
  IC1/1 -> Switch3/1
  Divide1/1 -> Relational Operator2/2
  Logical Operator2/1 -> Unit Delay/1, Switch/2
  Strt/1 -> Logical Operator2/2
  Unit Delay/1 -> Logical Operator2/1
  Switch/1 -> Sum/2
  Increment/1 -> Switch/1
  StopCounter/1 -> Switch/3
  RunnablePeriod/1 -> Divide/2
  Perd/1 -> Divide2/1, Divide/1

== system UXFD_Lib/CCM/Rate Limiter IC ==
  up : Inport  OutDataTypeStr=InputOutputDataType
  u : Inport  Port=2  OutDataTypeStr=InputOutputDataType
  IC : Inport  Port=3  OutDataTypeStr=InputOutputDataType
  T : Inport  Port=4  OutDataTypeStr=VCCTiSamplePerd
  lo : Inport  Port=5  OutDataTypeStr=InputOutputDataType
  Data Type Conversion{1..5} (5 alike) : DataTypeConversion  OutDataTypeStr=single  SaturateOnIntegerOverflow=on
  Difference Inputs1 : Sum  Description=Add in CPU  DisableCoverage=on  Inputs=+-  OutDataTypeStr=single  SaturateOnIntegerOverflow=on
  Difference Inputs2 : Sum  Description=Add in CPU  OutDataTypeStr=single  SaturateOnIntegerOverflow=on
  Saturation Dynamic : simulink/Discontinuities/Saturation Dynamic  OutMin=[]  OutMax=[]  OutDataTypeStr=single  OutputDataTypeScalingMode=single  OutDataType=dataType  OutScaling=[]  DoSatur=on
  Unit Delay External IC : CCMLib/Unit Delay External IC  dataType=single
  dataType : DataTypeConversion  OutDataTypeStr=InputOutputDataType  SaturateOnIntegerOverflow=on
  delta fall limit : Product  DisableCoverage=on  Inputs=**  OutDataTypeStr=single  SaturateOnIntegerOverflow=on
  delta rise limit : Product  DisableCoverage=on  Inputs=**  OutDataTypeStr=single  SaturateOnIntegerOverflow=on
  Y : Outport  OutDataTypeStr=InputOutputDataType  InitialOutput=0
  wires:
  dataType/1 -> Y/1
  Data Type Conversion4/1 -> delta fall limit/2
  Data Type Conversion3/1 -> Unit Delay External IC/2
  Data Type Conversion2/1 -> Difference Inputs1/1
  Data Type Conversion1/1 -> delta rise limit/1
  T/1 -> Data Type Conversion5/1
  lo/1 -> Data Type Conversion4/1
  delta rise limit/1 -> Saturation Dynamic/1
  up/1 -> Data Type Conversion1/1
  Difference Inputs2/1 -> dataType/1, Unit Delay External IC/1
  Unit Delay External IC/1 -> Difference Inputs1/2, Difference Inputs2/2
  Saturation Dynamic/1 -> Difference Inputs2/1
  delta fall limit/1 -> Saturation Dynamic/3
  u/1 -> Data Type Conversion2/1
  Difference Inputs1/1 -> Saturation Dynamic/2
  IC/1 -> Data Type Conversion3/1
  Data Type Conversion5/1 -> delta fall limit/1, delta rise limit/2

== system UXFD_Lib/CCM/Rate Limiter Resettable IC ==
  up : Inport  OutDataTypeStr=InputOutputDataType
  u : Inport  Port=2  OutDataTypeStr=InputOutputDataType
  IC : Inport  Port=3  OutDataTypeStr=InputOutputDataType
  T : Inport  Port=4  OutDataTypeStr=VCCTiSamplePerd
  lo : Inport  Port=5  OutDataTypeStr=InputOutputDataType
  R : Inport  Port=6  OutDataTypeStr=boolean
  Data Type Conversion{1..5} (5 alike) : DataTypeConversion  OutDataTypeStr=single  SaturateOnIntegerOverflow=on
  Difference Inputs1 : Sum  Description=Add in CPU  DisableCoverage=on  Inputs=+-  OutDataTypeStr=single  SaturateOnIntegerOverflow=on
  Difference Inputs2 : Sum  Description=Add in CPU  OutDataTypeStr=single  SaturateOnIntegerOverflow=on
  FixPt Data Type Duplicate : DataTypeDuplicate  DisableCoverage=on  NumInputPorts=7
  Saturation Dynamic : simulink/Discontinuities/Saturation Dynamic  OutMin=[]  OutMax=[]  OutDataTypeStr=single  OutputDataTypeScalingMode=single  OutDataType=dataType  OutScaling=[]  DoSatur=on
  Switch : Switch  Criteria=u2 ~= 0  SaturateOnIntegerOverflow=on
  Unit Delay Resettable External IC boolean controlled : Subsystem  mask(Unit Delay Resettable External Initial Condition (boolean)){dt=single, UnitDelayInitCondition=0}
      mask prompts: dt "Data type in/out"; UnitDelayInitCondition "Internal unit delay block initial condition:"
      mask help:
      | This is the same block as the Simulink standard, except all fix point
      | data-types have been changed to booleans.
      | The internal unit delay block can often be kept as 0, unless the input/output signal is of ENUM type.
      | Made by Niklas Magnusson (nmagnus3).
      | NGCC
      mask Display: dpoly(1,[1 0],'z')
  dataType : DataTypeConversion  OutDataTypeStr=InputOutputDataType  SaturateOnIntegerOverflow=on
  delta fall limit : Product  DisableCoverage=on  Inputs=**  OutDataTypeStr=single  SaturateOnIntegerOverflow=on
  delta rise limit : Product  DisableCoverage=on  Inputs=**  OutDataTypeStr=single  SaturateOnIntegerOverflow=on
  Y : Outport  OutDataTypeStr=InputOutputDataType  InitialOutput=0
  wires:
  Switch/1 -> dataType/1
  Data Type Conversion5/1 -> delta rise limit/2, delta fall limit/1
  R/1 -> Switch/2, Unit Delay Resettable External IC boolean controlled/2(R)
  IC/1 -> Data Type Conversion3/1
  Difference Inputs1/1 -> FixPt Data Type Duplicate/4, Saturation Dynamic/2
  u/1 -> Data Type Conversion2/1
  delta fall limit/1 -> FixPt Data Type Duplicate/3, Saturation Dynamic/3
  Saturation Dynamic/1 -> Difference Inputs2/1, FixPt Data Type Duplicate/7
  Unit Delay Resettable External IC boolean controlled/1(y) -> Difference Inputs2/2, Difference Inputs1/2, FixPt Data Type Duplicate/2
  Difference Inputs2/1 -> Switch/3, FixPt Data Type Duplicate/1, Unit Delay Resettable External IC boolean controlled/1(u)
  up/1 -> Data Type Conversion1/1
  delta rise limit/1 -> FixPt Data Type Duplicate/6, Saturation Dynamic/1
  lo/1 -> Data Type Conversion4/1
  T/1 -> Data Type Conversion5/1
  Data Type Conversion1/1 -> delta rise limit/1
  Data Type Conversion2/1 -> Difference Inputs1/1, FixPt Data Type Duplicate/5
  Data Type Conversion3/1 -> Switch/1, Unit Delay Resettable External IC boolean controlled/3(IC)
  Data Type Conversion4/1 -> delta fall limit/2
  dataType/1 -> Y/1

== system UXFD_Lib/CCM/SR_latch ==
  Set : Inport  OutDataTypeStr=boolean
  Reset : Inport  Port=2  OutDataTypeStr=boolean
  Logical Operator : Logic  AllPortsSameDT=off  OutDataTypeStr=boolean
  Logical Operator1 : Logic  Operator=OR  AllPortsSameDT=off  OutDataTypeStr=boolean
  Logical Operator2 : Logic  Operator=NOT  AllPortsSameDT=off  OutDataTypeStr=boolean
  Unit Delay External IC : simulink/Additional Math & Discrete/Additional Discrete/Unit Delay External IC  tsamp=-1
  false : Constant  Value=false  OutDataTypeStr=boolean  SampleTime=-1
  SetState : Outport  OutDataTypeStr=boolean
  wires:
  Set/1 -> Logical Operator1/2
  false/1 -> Unit Delay External IC/2
  Unit Delay External IC/1 -> Logical Operator1/1
  Logical Operator2/1 -> Logical Operator/2
  Reset/1 -> Logical Operator2/1
  Logical Operator1/1 -> Logical Operator/1
  Logical Operator/1 -> Unit Delay External IC/1, SetState/1

== system UXFD_Lib/CCM/SR_latch_NoRst ==
  Set : Inport  OutDataTypeStr=boolean
  Logical Operator1 : Logic  Operator=OR  AllPortsSameDT=off  OutDataTypeStr=boolean
  Unit Delay External IC : simulink/Additional Math & Discrete/Additional Discrete/Unit Delay External IC  tsamp=-1
  false : Constant  Value=false  OutDataTypeStr=boolean  SampleTime=-1
  SetState : Outport  OutDataTypeStr=boolean
  wires:
  Logical Operator1/1 -> SetState/1, Unit Delay External IC/1
  Unit Delay External IC/1 -> Logical Operator1/1
  false/1 -> Unit Delay External IC/2
  Set/1 -> Logical Operator1/2

== system UXFD_Lib/CCM/Timer ==
  note: CounterRunning
  note: If timer is set to zero, use start/hold/reset-status as output.
      | This is to avoid TimerFinished to be set to true without even the timer has started.
  Start : Inport  OutDataTypeStr=boolean
  Reset : Inport  Port=2  OutDataTypeStr=boolean
  Time : Inport  Port=3  OutDataTypeStr=timeDataType
  Divide : Product  Inputs=*/  OutDataTypeStr=VCCUInt32  RndMeth=Round  SaturateOnIntegerOverflow=on
  IC : Constant  Value=0  OutDataTypeStr=VCCUInt32  SampleTime=-1
  Increment : Constant  OutDataTypeStr=VCCUInt32  SampleTime=-1
  Logical Operator : Logic  AllPortsSameDT=off  OutDataTypeStr=boolean
  Logical Operator2 : Logic  Operator=OR  AllPortsSameDT=off  OutDataTypeStr=boolean
  Logical Operator3 : Logic  Operator=NOT  AllPortsSameDT=off  OutDataTypeStr=boolean
  Relational Operator : RelationalOperator  OutDataTypeStr=boolean  RndMeth=Nearest
  Relational Operator1 : RelationalOperator  Operator=>  OutDataTypeStr=boolean  RndMeth=Nearest
  RunnablePeriod : Constant  Value=RunnablePeriod  OutDataTypeStr=VCCTiSamplePerd  SampleTime=-1
  StopCounter : Constant  Value=0  OutDataTypeStr=VCCUInt32  SampleTime=-1
  Sum : Sum  OutDataTypeStr=VCCUInt32  SaturateOnIntegerOverflow=on
  Switch : Switch  Criteria=u2 ~= 0  SaturateOnIntegerOverflow=on
  Switch1 : Switch  Criteria=u2 ~= 0  SaturateOnIntegerOverflow=on
  Unit Delay External IC : simulink/Additional Math & Discrete/Additional Discrete/Unit Delay External IC  tsamp=-1
  Unit Delay Resettable External IC1 : CCMLib/Unit Delay Resettable External IC  dataType=VCCUInt32
  ZeroTicks : Constant  Value=0  OutDataTypeStr=VCCUInt32  SampleTime=-1
  false : Constant  Value=false  OutDataTypeStr=boolean  SampleTime=-1
  TimerFinished : Outport  OutDataTypeStr=boolean
  wires:
  Logical Operator2/1 -> Logical Operator/1
  false/1 -> Unit Delay External IC/2
  Logical Operator/1 -> Switch/2, Unit Delay External IC/1, Switch1/3
  Start/1 -> Logical Operator2/2
  Unit Delay External IC/1 -> Logical Operator2/1
  Unit Delay Resettable External IC1/1 -> Sum/1, Relational Operator/1
  Switch/1 -> Sum/2
  Increment/1 -> Switch/1
  StopCounter/1 -> Switch/3
  RunnablePeriod/1 -> Divide/2
  ZeroTicks/1 -> Relational Operator1/2
  Relational Operator1/1 -> Switch1/2
  Relational Operator/1 -> Switch1/1
  Divide/1 -> Relational Operator/2, Relational Operator1/1
  Switch1/1 -> TimerFinished/1
  Logical Operator3/1 -> Logical Operator/2
  Reset/1 -> Logical Operator3/1, Unit Delay Resettable External IC1/3
  Time/1 -> Divide/1
  IC/1 -> Unit Delay Resettable External IC1/2
  Sum/1 -> Unit Delay Resettable External IC1/1
